simulink library "DLE_tension_controller_v2"  (R2025b)
settings: Solver=VariableStepAuto  StartTime=0.0  StopTime=10.0  RelTol=1e-3
libraries: simulink x4, slpidlib x1
settings Model: Creator=cmmcguir  LastModifiedBy=cmmcguir

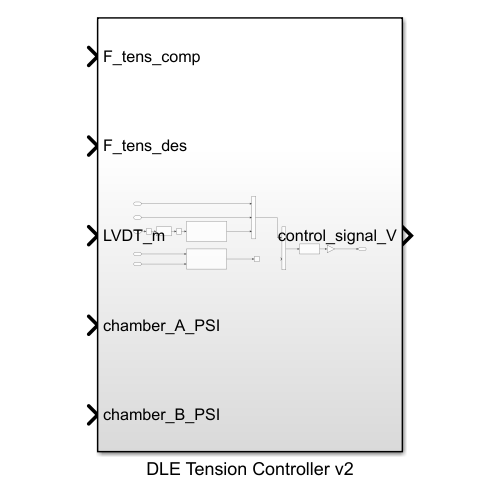
[thumbnail: Simulink's stored preview of the top-level diagram]
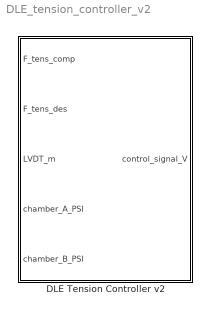
== system DLE_tension_controller_v2 ==
  DLE Tension Controller v2 : Subsystem

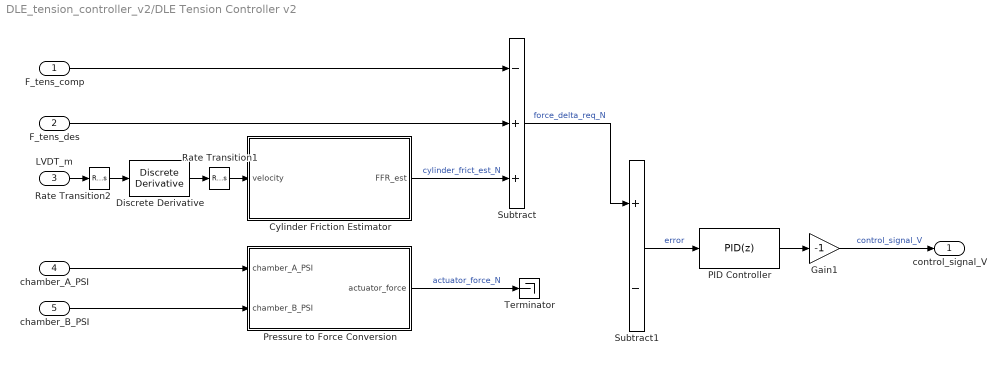
== system DLE_tension_controller_v2/DLE Tension Controller v2 ==
  F_tens_comp : Inport
  F_tens_des : Inport  Port=2
  LVDT_m : Inport  Port=3
  chamber_A_PSI : Inport  Port=4
  chamber_B_PSI : Inport  Port=5
  Cylinder Friction Estimator : Subsystem
  Discrete Derivative : simulink/Discrete/Discrete Derivative  gainval=1.0  ICPrevScaledInput=0.0  OutMin=[]  OutMax=[]  OutDataType=fixdt(1, 16)  OutScaling=2^-10  DoSatur=off
  Gain1 : Gain  Gain=-1
  PID Controller : slpidlib/PID Controller  Controller=PID  Form=Parallel  TimeDomain=Discrete-time  UseExternalTs=off  SampleTime=-1  IntegratorMethod=Forward Euler  FilterMethod=Forward Euler  ControllerParametersSource=internal  P=0.01  I=0.125*0  UseKiTs=off  D=0  UseExternalDerivativeSource=off  N=100  UseFilter=on  TunerSelectOption=Transfer Function Based (PID Tuner App)  InitialConditionSource=internal  InitialConditionForIntegrator=0  InitialConditionForFilter=0  DifferentiatorICPrevScaledInput=0  ExternalReset=none  TrackingMode=off  Kt=1  LimitOutput=on  SatLimitsSource=internal  UpperSaturationLimit=10  LowerSaturationLimit=-10  LinearizeAsGain=off  AntiWindupMode=clamping  Kb=1  LimitIntegrator=off  UpperIntegratorSaturationLimit=inf  LowerIntegratorSaturationLimit=-inf  POutMin=[]  POutMax=[]  IOutMin=[]  IOutMax=[]  DOutMin=[]  DOutMax=[]  NOutMin=[]  NOutMax=[]  SumOutMin=[]  SumOutMax=[]  SaturationOutMin=[]  SaturationOutMax=[]  PParamMin=[]  PParamMax=[]  IParamMin=[]  IParamMax=[]  DParamMin=[]  DParamMax=[]  NParamMin=[]  NParamMax=[]  KbParamMin=[]  KbParamMax=[]  KtParamMin=[]  KtParamMax=[]  KbOutMin=[]  KbOutMax=[]  KtOutMin=[]  KtOutMax=[]  IntegratorOutMin=[]  IntegratorOutMax=[]  FilterOutMin=[]  FilterOutMax=[]  SumI1OutMin=[]  SumI1OutMax=[]  SumI2OutMin=[]  SumI2OutMax=[]  SumI3OutMin=[]  SumI3OutMax=[]  SumI4OutMin=[]  SumI4OutMax=[]  SumDOutMin=[]  SumDOutMax=[]  DifferentiatorOutMin=[]  DifferentiatorOutMax=[]  FilterDiffOutCoefMin=[]  FilterDiffOutCoefMax=[]  ReciprocalOutMin=[]  ReciprocalOutMax=[]  SumDenOutMin=[]  SumDenOutMax=[]  SumNumOutMin=[]  SumNumOutMax=[]  DivideOutMin=[]  DivideOutMax=[]  UdiffTsProdOutMin=[]  UdiffTsProdOutMax=[]  NTsProdOutMin=[]  NTsProdOutMax=[]  UintegralTsProdOutMin=[]  UintegralTsProdOutMax=[]  UngainTsProdOutMin=[]  UngainTsProdOutMax=[]  ClampingZeroOutDataTypeStr=Inherit: Inherit via back propagation  ClampingZeroOutMin=[]  ClampingZeroOutMax=[]  FilterDenConstantOutDataTypeStr=Inherit: Inherit via back propagation  FilterDenConstantOutMin=[]  FilterDenConstantOutMax=[]  PCopyOutDataTypeStr=Inherit: Inherit via back propagation  PCopyOutMin=[]  PCopyOutMax=[]  NCopyOutDataTypeStr=Inherit: Inherit via back propagation  NCopyOutMin=[]  NCopyOutMax=[]  IntegratorContinuousStateAttributes=''  IntegratorStateMustResolveToSignalObject=off  IntegratorRTWStateStorageClass=Auto  FilterContinuousStateAttributes=''  FilterStateMustResolveToSignalObject=off  FilterRTWStateStorageClass=Auto  ParallelPVariant=InternalParameters  IdealPVariant=Disabled  IVariant=InternalParameters  DVariant=InternalParameters  IntegratorVariant=Discrete  SatVariant=Enabled  AWVariant=DiscClampingParallel  PCopyVariant=Disabled  TRVariant=Disabled  FdbkBlocksVariant=Forward  IdealPFdbkVariant=Disabled  SatFdbkVariant=Disabled  DerivativeFilterVariant=ForwardEulerFilter  NVariant=InternalParameters  NCopyVariant=Disabled  FilterICVariant=InternalICsFilter  IntegratorICVariant=InternalICs  ExternalResetVariant=Disabled  TRSumVariant=Passthrough  SumFdbkVariant=Disabled  SumVariant=Sum_PID  TsampFilterVariant=InternalTs  TsampNgainVariant=Passthrough  TsampIntegralVariant=Disabled_SignalSpec  ExternalSaturationOutDataTypeStr=Inherit: Same as second input  DerivativeSourceVariant=ErrorSignal  PreIntVariant=InternalPreInt
  Pressure to Force Conversion : Subsystem
  Rate Transition1 : RateTransition  OutPortSampleTime=0.0001
  Rate Transition2 : RateTransition  OutPortSampleTime=0.001
  Subtract : Sum  Inputs=-++
  Subtract1 : Sum  Inputs=+-
  Terminator : Terminator
  control_signal_V : Outport
  wires:
  chamber_A_PSI/1 -> Pressure to Force Conversion/1(chamber_A_PSI)
  chamber_B_PSI/1 -> Pressure to Force Conversion/2(chamber_B_PSI)
  Discrete Derivative/1 -> Rate Transition1/1
  LVDT_m/1 -> Rate Transition2/1
  Cylinder Friction Estimator/1(FFR_est) -> Subtract/3  "cylinder_frict_est_N"
  F_tens_comp/1 -> Subtract/1
  Subtract/1 -> Subtract1/1  "force_delta_req_N"
  Pressure to Force Conversion/1(actuator_force) -> Terminator/1  "actuator_force_N"
  Subtract1/1 -> PID Controller/1  "error"
  PID Controller/1 -> Gain1/1
  Rate Transition2/1 -> Discrete Derivative/1
  Rate Transition1/1 -> Cylinder Friction Estimator/1(velocity)
  F_tens_des/1 -> Subtract/2
  Gain1/1 -> control_signal_V/1  "control_signal_V"

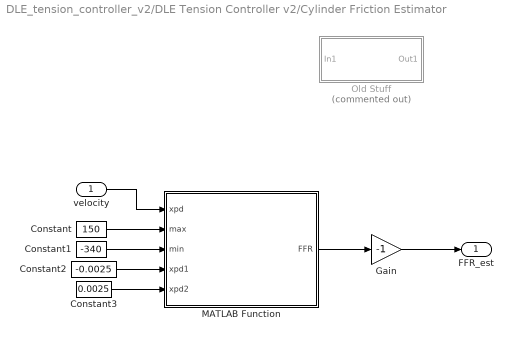
== system DLE_tension_controller_v2/DLE Tension Controller v2/Cylinder Friction Estimator ==
  velocity : Inport
  Constant : Constant  Value=150
  Constant1 : Constant  Value=-340
  Constant2 : Constant  Value=-0.0025
  Constant3 : Constant  Value=0.0025
  Gain : Gain  Gain=-1
  MATLAB Function : MATLAB Function  TreatAsAtomicUnit=on
  Old Stuff : Subsystem  Commented=on
  FFR_est : Outport  VectorParamsAs1DForOutWhenUnconnected=off
  wires:
  Constant/1 -> MATLAB Function/2(max)
  Constant1/1 -> MATLAB Function/3(min)
  Constant2/1 -> MATLAB Function/4(xpd1)
  Constant3/1 -> MATLAB Function/5(xpd2)
  velocity/1 -> MATLAB Function/1(xpd)
  MATLAB Function/1(FFR) -> Gain/1
  Gain/1 -> FFR_est/1

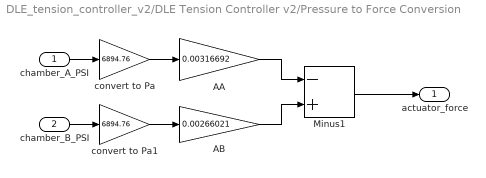
== system DLE_tension_controller_v2/DLE Tension Controller v2/Pressure to Force Conversion ==
  chamber_A_PSI : Inport
  chamber_B_PSI : Inport  Port=2
  AA : Gain  Gain=0.00316692
  AB : Gain  Gain=0.00266021
  Minus1 : Sum  Inputs=-+
  convert to Pa : Gain  Gain=6894.76
  convert to Pa1 : Gain  Gain=6894.76
  actuator_force : Outport  VectorParamsAs1DForOutWhenUnconnected=off
  wires:
  Minus1/1 -> actuator_force/1
  convert to Pa/1 -> AA/1
  AA/1 -> Minus1/1
  convert to Pa1/1 -> AB/1
  AB/1 -> Minus1/2
  chamber_A_PSI/1 -> convert to Pa/1
  chamber_B_PSI/1 -> convert to Pa1/1

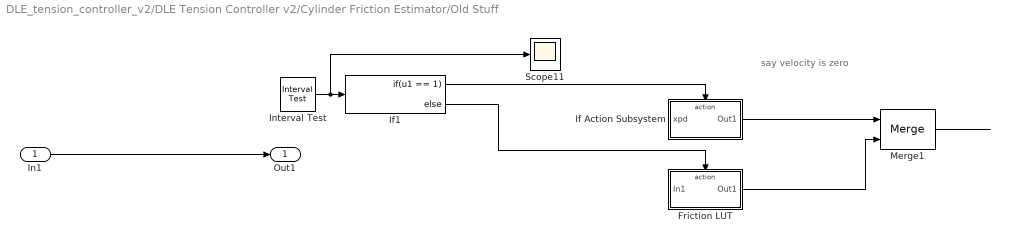
== system DLE_tension_controller_v2/DLE Tension Controller v2/Cylinder Friction Estimator/Old Stuff ==
  note: say velocity is zero
  In1 : Inport
  Friction LUT : Subsystem  TreatAsAtomicUnit=on
  If Action Subsystem : Subsystem  TreatAsAtomicUnit=on
  If1 : If  IfExpression=u1 == 1
  Interval Test : simulink/Logic and Bit Operations/Interval Test  IntervalClosedRight=on  uplimit=0.006  IntervalClosedLeft=on  lowlimit=-0.004  OutDataTypeStr=boolean
  Merge1 : Merge
  Scope11 : Scope
      settings: ActiveDisplayYMinimum=-0.125  ActiveDisplayYMaximum=1.125
  Out1 : Outport  VectorParamsAs1DForOutWhenUnconnected=off
  wires:
  In1/1 -> Out1/1
  If1/2 -> Friction LUT/Action
  ? -> If Action Subsystem/1(xpd), Interval Test/1
  If1/1 -> If Action Subsystem/Action
  ? -> Friction LUT/1(In1)
  If Action Subsystem/1(Out1) -> Merge1/1
  Friction LUT/1(Out1) -> Merge1/2
  Interval Test/1 -> If1/1, Scope11/1
  Merge1/1 -> ?

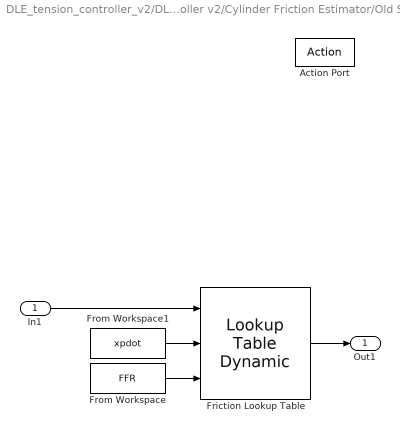
== system DLE_tension_controller_v2/DLE Tension Controller v2/Cylinder Friction Estimator/Old Stuff/Friction LUT ==
  In1 : Inport
  Action Port : ActionPort
  Friction Lookup Table : simulink/Lookup Tables/Lookup Table Dynamic  LookUpMeth=Interpolation-Use End Values  OutDataType=fixdt('double')  OutScaling=[]  OutputDataTypeScalingMode=Specify via dialog  OutDataTypeStr=double  DoSatur=off
  From Workspace : FromWorkspace  VariableName=FFR
  From Workspace1 : FromWorkspace  VariableName=xpdot
  Out1 : Outport  VectorParamsAs1DForOutWhenUnconnected=off
  wires:
  From Workspace1/1 -> Friction Lookup Table/2
  From Workspace/1 -> Friction Lookup Table/3
  In1/1 -> Friction Lookup Table/1
  Friction Lookup Table/1 -> Out1/1

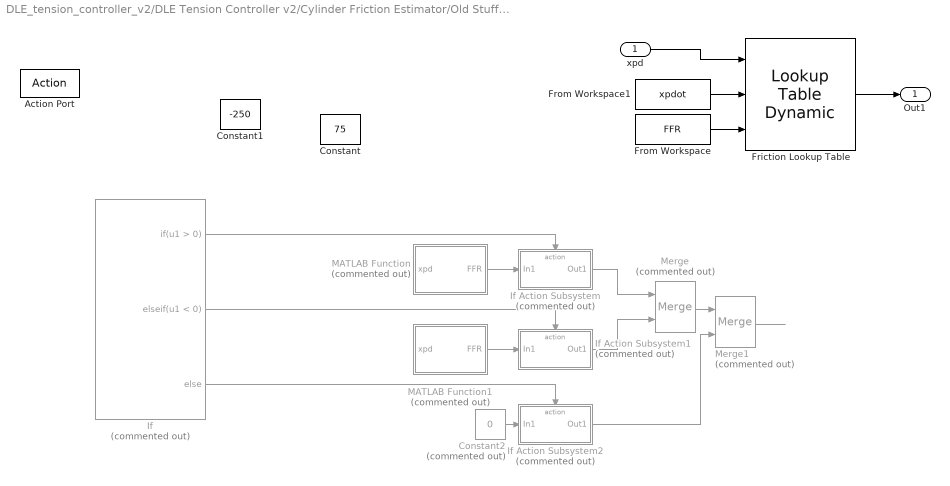
== system DLE_tension_controller_v2/DLE Tension Controller v2/Cylinder Friction Estimator/Old Stuff/If Action Subsystem ==
  xpd : Inport
  Action Port : ActionPort
  Constant : Constant  Value=75
  Constant1 : Constant  Value=-250
  Constant2 : Constant  Commented=on  Value=0
  Friction Lookup Table : simulink/Lookup Tables/Lookup Table Dynamic  LookUpMeth=Interpolation-Use End Values  OutDataType=fixdt('double')  OutScaling=[]  OutputDataTypeScalingMode=Specify via dialog  OutDataTypeStr=double  DoSatur=off
  From Workspace : FromWorkspace  VariableName=FFR
  From Workspace1 : FromWorkspace  VariableName=xpdot
  If : If  Commented=on  ElseIfExpressions=u1 < 0
  If Action Subsystem : Subsystem  Commented=on  TreatAsAtomicUnit=on
  If Action Subsystem1 : Subsystem  Commented=on  TreatAsAtomicUnit=on
  If Action Subsystem2 : Subsystem  Commented=on  TreatAsAtomicUnit=on
  MATLAB Function : MATLAB Function  Commented=on  TreatAsAtomicUnit=on
  MATLAB Function1 : MATLAB Function  Commented=on  TreatAsAtomicUnit=on
  Merge : Merge  Commented=on
  Merge1 : Merge  Commented=on
  Out1 : Outport  VectorParamsAs1DForOutWhenUnconnected=off
  wires:
  Friction Lookup Table/1 -> Out1/1
  xpd/1 -> Friction Lookup Table/1
  From Workspace/1 -> Friction Lookup Table/3
  From Workspace1/1 -> Friction Lookup Table/2
  ? -> MATLAB Function/1(xpd), MATLAB Function1/1(xpd), If/1
  If Action Subsystem/1(Out1) -> Merge/1
  MATLAB Function/1(FFR) -> If Action Subsystem/1(In1)
  If/2 -> If Action Subsystem1/Action
  If Action Subsystem1/1(Out1) -> Merge/2
  If/1 -> If Action Subsystem/Action
  If/3 -> If Action Subsystem2/Action
  Merge/1 -> Merge1/1
  Merge1/1 -> ?
  If Action Subsystem2/1(Out1) -> Merge1/2
  Constant2/1 -> If Action Subsystem2/1(In1)
  MATLAB Function1/1(FFR) -> If Action Subsystem1/1(In1)

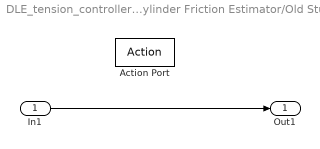
== system DLE_tension_controller_v2/DLE Tension Controller v2/Cylinder Friction Estimator/Old Stuff/If Action Subsystem/If Action Subsystem ==
  In1 : Inport
  Action Port : ActionPort
  Out1 : Outport  VectorParamsAs1DForOutWhenUnconnected=off
  wires:
  In1/1 -> Out1/1

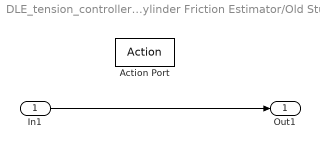
== system DLE_tension_controller_v2/DLE Tension Controller v2/Cylinder Friction Estimator/Old Stuff/If Action Subsystem/If Action Subsystem1 ==
  In1 : Inport
  Action Port : ActionPort
  Out1 : Outport  VectorParamsAs1DForOutWhenUnconnected=off
  wires:
  In1/1 -> Out1/1

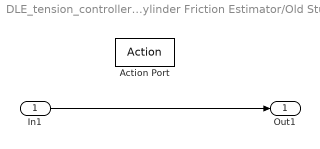
== system DLE_tension_controller_v2/DLE Tension Controller v2/Cylinder Friction Estimator/Old Stuff/If Action Subsystem/If Action Subsystem2 ==
  In1 : Inport
  Action Port : ActionPort
  Out1 : Outport  VectorParamsAs1DForOutWhenUnconnected=off
  wires:
  In1/1 -> Out1/1

== matlab function DLE_tension_controller_v2/DLE Tension Controller v2/Cylinder Friction Estimator/Old Stuff/If Action Subsystem/MATLAB Function ==
  data: xpd input; FFR output
function FFR = fcn(xpd)

FFR = 250/0.006*xpd; %linear fit for static friction force
end

== matlab function DLE_tension_controller_v2/DLE Tension Controller v2/Cylinder Friction Estimator/Old Stuff/If Action Subsystem/MATLAB Function1 ==
  data: xpd input; FFR output
function FFR = fcn(xpd)

FFR = 450/0.004*xpd; %linear fit for static friction force
end

== matlab function DLE_tension_controller_v2/DLE Tension Controller v2/Cylinder Friction Estimator/MATLAB Function ==
  data: xpd input; FFR output; max input; min input; xpd1 input; xpd2 input
function FFR = FrictionPoly(xpd, max, min,xpd1, xpd2)

p_pos = [286259495.429843,-173193752.694681,41175113.3821288,-4870042.97579715,308159.025845462,-8434.36139981410,146.161974739502];
p_neg = [-162371605.890866,-93401901.1521574,-21487354.7937511,-2556477.89021572,-183283.452954630,-6357.37685861595,-310.459473151221];


if xpd > xpd2
        
        if xpd <= 0.179334
            FFR = polyval(p_pos, xpd); %positive friction curve
        else
%             FFR = 3828.541*xpd - 249.1766; %linear extrapolation past what I have
                FFR = polyval(p_pos, .179334);
        end
    
elseif xpd < xpd1

        if xpd >= -0.1648
            FFR = polyval(p_neg, xpd); %negative friction curve
        else
%             FFR = 3211*xpd - 7.106;
                FFR = polyval(p_neg, -0.1648);
        end    
else
    

    FFR1 = polyval(p_neg, xpd1);
    FFR2 = polyval(p_pos, xpd2);

% FFR1 = min;
% FFR2 = max;
    
    FFR = interp1([xpd1 xpd2],[FFR1, FFR2], xpd);
% FFR = 0;
%     if xpdd > 0 %if concavity is positive
% %         
%        FFR = -350; %positive friction curve
% %        
%     elseif xpdd < 0
% % 
%         FFR = 150; %negative friction curve
%         
%     else
%         
%         FFR = 0;
%         
%     end

end

end
